simulink model "BT_da_train_cach2"  (R2017b)
settings: Solver=ode5  StartTime=0.0  StopTime=60  FixedStep=0.01  RelTol=1e-3
libraries: neural x305, powerlib_meascontrol x1
(part 4 of 4)

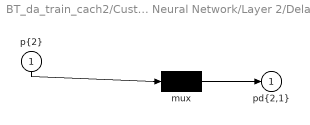
== system BT_da_train_cach2/Custom Neural Network/Layer 2/Delays 1 ==
  "p{2}" : Inport  PortDimensions=300
      mask Display: e = 0.06;c1 = [120 230 180]/255;c2 = ([120 230 180]+0)/(256+128);c3 = ([120 230 180]+128)/(256+128);patch([0 1 1 0],[0 0 1 1],c1);patch([0 1 1 1-e 1-e 0+e],[0 0 1 1-e 0+e 0+e],c2);patch([0 0 1 1-e 0+e 0+e],[0 1 1 1-e 1-e 0+e],c3);plot([0 1 1 0 0],[0 0 1 1 0]);
  mux : Mux  Inputs=1
      mask Display: e = 0.06;c1 = [120 150 230]/255;c2 = ([120 150 230]+0)/383;c3 = ([120 150 230]+128)/383;patch([0 1 1 0],[0 0 1 1],c1);patch([0 1 1 1-e 1-e 0+e],[0 0 1 1-e 0+e 0+e],c2);patch([0 0 1 1-e 0+e 0+e],[0 1 1 1-e 1-e 0+e],c3);plot([0 1 1 0 0],[0 0 1 1 0]);disp('Mux')
  "pd{2,1}" : Outport
      mask Display: e = 0.06;c1 = [120 230 180]/255;c2 = ([120 230 180]+0)/(256+128);c3 = ([120 230 180]+128)/(256+128);patch([0 1 1 0],[0 0 1 1],c1);patch([0 1 1 1-e 1-e 0+e],[0 0 1 1-e 0+e 0+e],c2);patch([0 0 1 1-e 0+e 0+e],[0 1 1 1-e 1-e 0+e],c3);plot([0 1 1 0 0],[0 0 1 1 0]);
  wires:
  "p{2}"/1 -> mux/1
  mux/1 -> "pd{2,1}"/1

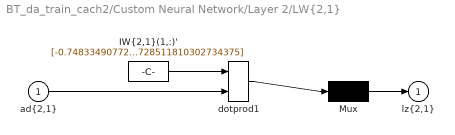
== system BT_da_train_cach2/Custom Neural Network/Layer 2/LW{2,1} ==
  "ad{2,1}" : Inport  PortDimensions=300
      mask Display: e = 0.06;c1 = [120 230 180]/255;c2 = ([120 230 180]+0)/(256+128);c3 = ([120 230 180]+128)/(256+128);patch([0 1 1 0],[0 0 1 1],c1);patch([0 1 1 1-e 1-e 0+e],[0 0 1 1-e 0+e 0+e],c2);patch([0 0 1 1-e 0+e 0+e],[0 1 1 1-e 1-e 0+e],c3);plot([0 1 1 0 0],[0 0 1 1 0]);
  "IW{2,1}(1,:)'" : Constant  Value=[-0.7483349077278134142687804342131130397319793701171875;0.42689576643265436661778267080080695450305938720703125;0.43741311676930461072032585434499196708202362060546875;-0.392833763188094764462476859989692457020282745361328125;0.587520578048666752835060833604075014591217041015625;-0.69105477162133455149017891017138026654720306396484375;0.42810845242557871159760907175950706005096435546875;0.52490020256978631163491400002385489642620086669921875;-0.83551425158135106396883884372073225677013397216796875;-0.250808962743687635654765699655399657785892486572265625;-0.62072659871463364833488185468013398349285125732421875;0.1343949448524652534597834119267645291984081268310546875;0.525260239270437079284192805062048137187957763671875;0.10948844837812503338891900739326956681907176971435546875;-0.579867883609712198023089513299055397510528564453125;-0.442938627596811296260881363195949234068393707275390625;-0.56889662745070823657300707054673694074153900146484375;-0.1278602170445769792284096411094651557505130767822265625;-0.365421241431190868542699945464846678078174591064453125;-0.6343149410650730235516903121606446802616119384765625;-0.443920889039115695862136590221780352294445037841796875;-0.5821977817375165731306196903460659086704254150390625;-0.5678870795060693144051811032113619148731231689453125;0.244166050903289966189646520433598197996616363525390625;-0.422872158456276958649056041394942440092563629150390625;0.7905267869644092559866521696676500141620635986328125;-0.3162229010638684112421969985007308423519134521484375;-0.2048038452942719522820169686383451335132122039794921875;-0.21781996446133267131273214545217342674732208251953125;-0.192062904462992178888924854618380777537822723388671875;-0.116542569790399841433981009686249308288097381591796875;0.76972691893932176920856136348447762429714202880859375;-1.0542421909336230356757369008846580982208251953125;0.274235589667554513493286094671930186450481414794921875;0.91430233093692525603302101444569416344165802001953125;0.5391672295754397215006292753969319164752960205078125;0.1849346990733304607612552672435413114726543426513671875;-0.0176570878712307526015035108457595924846827983856201171875;-0.8913799022242281377970130051835440099239349365234375;0.515211847795638444580390569171868264675140380859375;0.1916727100862337385134281930731958709657192230224609375;-0.10443782149983125984160636789965792559087276458740234375;0.72574255400356124656724432497867383062839508056640625;-0.5440114992671680749225515683065168559551239013671875;0.492231731056198551499392124242149293422698974609375;-0.59763974029317090685964330987189896404743194580078125;0.1540445637943870516028965766963665373623371124267578125;-0.317467853625854556920415916465572081506252288818359375;0.488021785104874539218400286699761636555194854736328125;0.92569708577502429758254720582044683396816253662109375;0.338332780718257730701026275710319168865680694580078125;-0.681470581082837423281262090313248336315155029296875;-0.1254385107127151954831134617052157409489154815673828125;-0.287493825736406416471169222859316505491733551025390625;-0.2347218393909844547096099631744436919689178466796875;-0.2892408551971872299191090860404074192047119140625;0.8117439457287414228403576998971402645111083984375;0.1282227716762665281624578028640826232731342315673828125;0.30643388849748431912445312264026142656803131103515625;0.38498495598662041405901845791959203779697418212890625;-0.54251146855425369519565492737456224858760833740234375;-0.1701558644881129012116360854633967392146587371826171875;-0.7088895239048420560123986433609388768672943115234375;-0.662009407482496481378575481357984244823455810546875;0.296902088504847838645872570850769989192485809326171875;0.79351616015326087438808144725044257938861846923828125;-0.2304607186051676748217431622833828441798686981201171875;-1.089284272480465887156242388300597667694091796875;-0.192529255099039231513557979269535280764102935791015625;0.360627416201959205555027665468514896929264068603515625 ...(+13044 chars)]
      mask Display: e = 0.06;c1 = [120 150 230]/255;c2 = ([120 150 230]+0)/383;c3 = ([120 150 230]+128)/383;patch([0 1 1 0],[0 0 1 1],c1);patch([0 1 1 1-e 1-e 0+e],[0 0 1 1-e 0+e 0+e],c2);patch([0 0 1 1-e 0+e 0+e],[0 1 1 1-e 1-e 0+e],c3);plot([0 1 1 0 0],[0 0 1 1 0]);disp('weights');
  Mux : Mux  Inputs=1
      mask Display: e = 0.06;c1 = [120 150 230]/255;c2 = ([120 150 230]+0)/383;c3 = ([120 150 230]+128)/383;patch([0 1 1 0],[0 0 1 1],c1);patch([0 1 1 1-e 1-e 0+e],[0 0 1 1-e 0+e 0+e],c2);patch([0 0 1 1-e 0+e 0+e],[0 1 1 1-e 1-e 0+e],c3);plot([0 1 1 0 0],[0 0 1 1 0]);disp('Mux');
  dotprod1 : neural/Weight Functions/dotprod
  "lz{2,1}" : Outport
      mask Display: e = 0.06;c1 = [120 230 180]/255;c2 = ([120 230 180]+0)/(256+128);c3 = ([120 230 180]+128)/(256+128);patch([0 1 1 0],[0 0 1 1],c1);patch([0 1 1 1-e 1-e 0+e],[0 0 1 1-e 0+e 0+e],c2);patch([0 0 1 1-e 0+e 0+e],[0 1 1 1-e 1-e 0+e],c3);plot([0 1 1 0 0],[0 0 1 1 0]);
  wires:
  "IW{2,1}(1,:)'"/1 -> dotprod1/1
  "ad{2,1}"/1 -> dotprod1/2
  dotprod1/1 -> Mux/1
  Mux/1 -> "lz{2,1}"/1
